simulink model "small_perturbation_linearized_model_v2"  (R2019b)
settings: Solver=ode4  StartTime=0.0  StopTime=20  FixedStep=1e-3
settings Model: Creator=bitgar  LastModifiedBy=zczhu

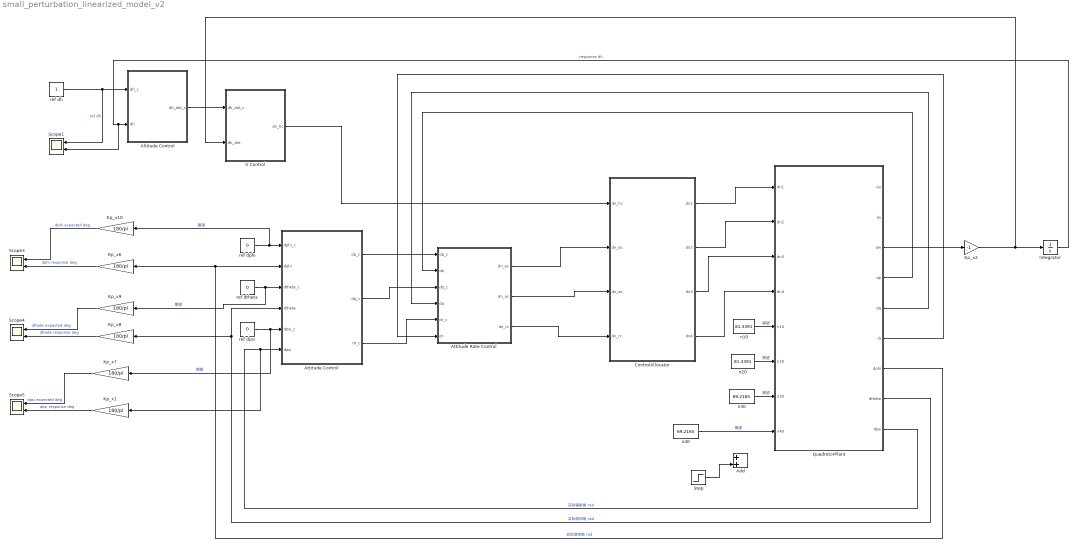
== system small_perturbation_linearized_model_v2 ==
  Add : Sum
  Altitude Control : Subsystem
  Attitude Control : Subsystem
  Attitude Rate Control : Subsystem
  ControlAllocator : Subsystem
  Integrator : Integrator
  Kp_x{1,6..10} (6 alike) : Gain  Gain=180/pi
  Kp_x2 : Gain  Gain=-1
  QuadrotorPlant : Subsystem
  Scope{1,3..5} (4 alike) : Scope  NumInputPorts=2
  Step : Step  Time=5  After=20  SampleTime=0
  V Control : Subsystem
  n10 : Constant  Value=81.3391
  n20 : Constant  Value=81.3391
  n30 : Constant  Value=69.2165
  n40 : Constant  Value=69.2165
  ref dh : Constant
  ref dphi : Constant  Value=0
  ref dpsi : Constant  Value=0
  ref dtheta : Constant  Value=0
  wires:
  Attitude Control/2(dq_c) -> Attitude Rate Control/3(dq_c)
  Attitude Control/1(dp_c) -> Attitude Rate Control/1(dp_c)
  ref dpsi/1 -> Kp_x7/1, Attitude Control/5(dpsi_c)  "期望"
  Attitude Rate Control/2(dn_ac) -> ControlAllocator/3(dn_ac)
  Attitude Rate Control/1(dn_ec) -> ControlAllocator/2(dn_ec)
  Attitude Rate Control/3(dn_rc) -> ControlAllocator/4(dn_rc)
  Attitude Control/3(dr_c) -> Attitude Rate Control/5(dr_c)
  Kp_x6/1 -> Scope3/2  "dphi response deg"
  Kp_x8/1 -> Scope4/2  "dtheta response deg"
  ControlAllocator/2(dn2) -> QuadrotorPlant/2(dn2)
  ControlAllocator/3(dn3) -> QuadrotorPlant/3(dn3)
  ControlAllocator/4(dn4) -> QuadrotorPlant/4(dn4)
  QuadrotorPlant/4(dp) -> Attitude Rate Control/2(dp)
  QuadrotorPlant/5(dq) -> Attitude Rate Control/4(dq)
  QuadrotorPlant/6(dr) -> Attitude Rate Control/6(dr)
  QuadrotorPlant/7(dphi) -> Kp_x6/1, Attitude Control/2(dphi)  "实际滚转角 rad"
  QuadrotorPlant/8(dtheta) -> Kp_x8/1, Attitude Control/4(dtheta)  "实际俯仰角 rad"
  QuadrotorPlant/9(dpsi) -> Kp_x1/1, Attitude Control/6(dpsi)  "实际偏航角 rad"
  ref dphi/1 -> Kp_x10/1, Attitude Control/1(dphi_c)  "期望"
  ref dtheta/1 -> Kp_x9/1, Attitude Control/3(dtheta_c)  "期望"
  n10/1 -> QuadrotorPlant/5(n10)  "期望"
  n20/1 -> QuadrotorPlant/6(n20)  "期望"
  n30/1 -> QuadrotorPlant/7(n30)  "期望"
  Kp_x1/1 -> Scope5/2  "dpsi response deg"
  Kp_x7/1 -> Scope5/1  "dpsi expected deg"
  Kp_x9/1 -> Scope4/1  "dtheta expected deg"
  Kp_x10/1 -> Scope3/1  "dphi expected deg"
  ControlAllocator/1(dn1) -> QuadrotorPlant/1(dn1)
  Step/1 -> Add/2
  ref dh/1 -> Scope1/1, Altitude Control/1(dh_c)  "ref dh"
  Altitude Control/1(dh_dot_c) -> V Control/1(dh_dot_c)
  V Control/1(dn_hc) -> ControlAllocator/1(dn_hc)
  QuadrotorPlant/3(dw) -> Kp_x2/1
  Integrator/1 -> Scope1/2, Altitude Control/2(dh)  "response dh"
  Kp_x2/1 -> V Control/2(dh_dot), Integrator/1
  n40/1 -> QuadrotorPlant/8(n40)  "期望"

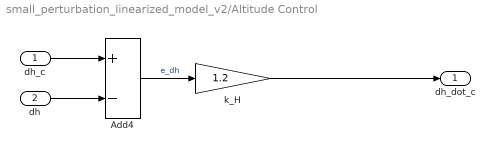
== system small_perturbation_linearized_model_v2/Altitude Control ==
  dh_c : Inport
  dh : Inport  Port=2
  Add4 : Sum  Inputs=+-
  k_H : Gain  Gain=1.2
  dh_dot_c : Outport
  wires:
  dh_c/1 -> Add4/1
  dh/1 -> Add4/2
  Add4/1 -> k_H/1  "e_dh"
  k_H/1 -> dh_dot_c/1

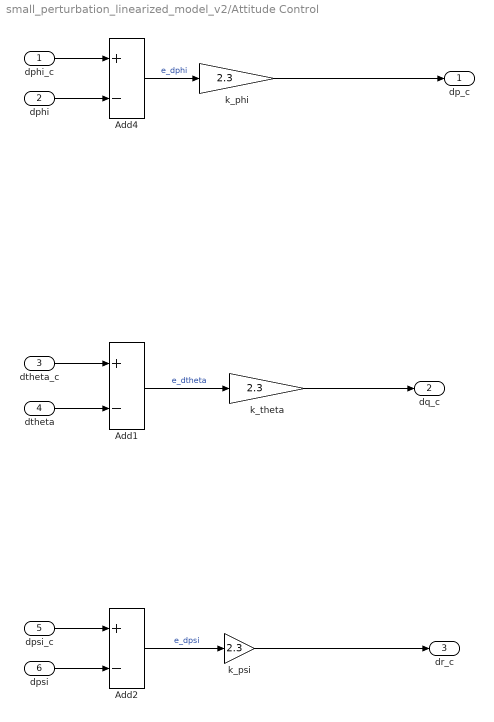
== system small_perturbation_linearized_model_v2/Attitude Control ==
  dphi_c : Inport
  dphi : Inport  Port=2
  dtheta_c : Inport  Port=3
  dtheta : Inport  Port=4
  dpsi_c : Inport  Port=5
  dpsi : Inport  Port=6
  Add1 : Sum  Inputs=+-
  Add2 : Sum  Inputs=+-
  Add4 : Sum  Inputs=+-
  k_phi : Gain  Gain=2.3
  k_psi : Gain  Gain=2.3
  k_theta : Gain  Gain=2.3
  dp_c : Outport
  dq_c : Outport  Port=2
  dr_c : Outport  Port=3
  wires:
  dphi_c/1 -> Add4/1
  dphi/1 -> Add4/2
  dtheta_c/1 -> Add1/1
  dtheta/1 -> Add1/2
  dpsi/1 -> Add2/2
  Add4/1 -> k_phi/1  "e_dphi"
  dpsi_c/1 -> Add2/1
  Add1/1 -> k_theta/1  "e_dtheta"
  Add2/1 -> k_psi/1  "e_dpsi"
  k_phi/1 -> dp_c/1
  k_theta/1 -> dq_c/1
  k_psi/1 -> dr_c/1

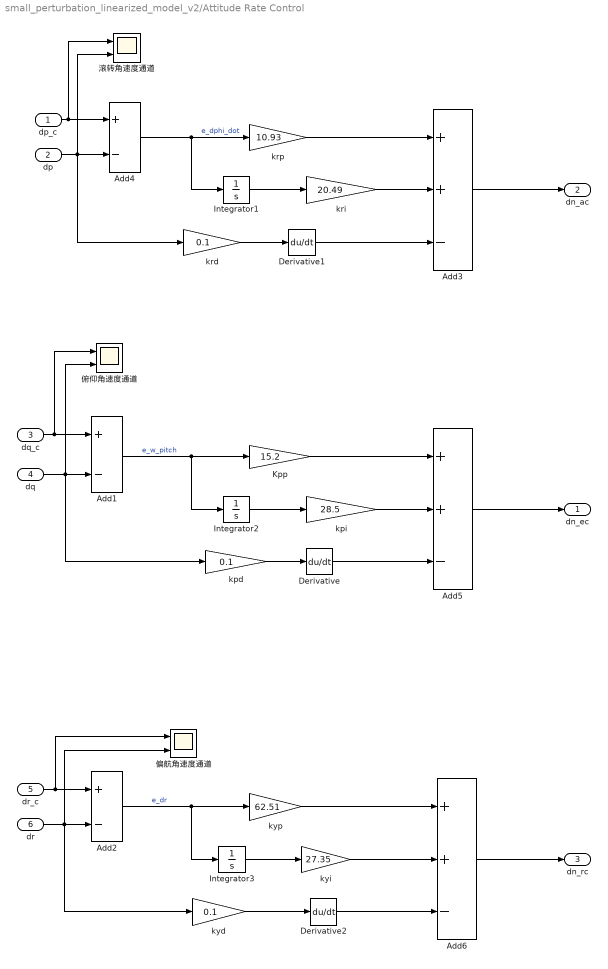
== system small_perturbation_linearized_model_v2/Attitude Rate Control ==
  dp_c : Inport
  dp : Inport  Port=2
  dq_c : Inport  Port=3
  dq : Inport  Port=4
  dr_c : Inport  Port=5
  dr : Inport  Port=6
  Add1 : Sum  Inputs=+-
  Add2 : Sum  Inputs=+-
  Add3 : Sum  Inputs=++-
  Add4 : Sum  Inputs=+-
  Add5 : Sum  Inputs=++-
  Add6 : Sum  Inputs=++-
  Derivative : Derivative
  Derivative1 : Derivative
  Derivative2 : Derivative
  Integrator1 : Integrator
  Integrator2 : Integrator
  Integrator3 : Integrator
  Kpp : Gain  Gain=15.2
  kpd : Gain  Gain=0.1
  kpi : Gain  Gain=28.5
  krd : Gain  Gain=0.1
  kri : Gain  Gain=20.49
  krp : Gain  Gain=10.93
  kyd : Gain  Gain=0.1
  kyi : Gain  Gain=27.35
  kyp : Gain  Gain=62.51
  俯仰角速度通道 : Scope  NumInputPorts=2
  偏航角速度通道 : Scope  NumInputPorts=2
  滚转角速度通道 : Scope  NumInputPorts=2
  dn_ec : Outport
  dn_ac : Outport  Port=2
  dn_rc : Outport  Port=3
  wires:
  dp_c/1 -> 滚转角速度通道/1, Add4/1
  dp/1 -> krd/1, 滚转角速度通道/2, Add4/2
  dq_c/1 -> 俯仰角速度通道/1, Add1/1
  dq/1 -> kpd/1, 俯仰角速度通道/2, Add1/2
  dr/1 -> 偏航角速度通道/2, kyd/1, Add2/2
  Add4/1 -> Integrator1/1, krp/1  "e_dphi_dot"
  dr_c/1 -> 偏航角速度通道/1, Add2/1
  Add3/1 -> dn_ac/1
  kri/1 -> Add3/2
  krp/1 -> Add3/1
  Integrator1/1 -> kri/1
  Integrator2/1 -> kpi/1
  Kpp/1 -> Add5/1
  kpi/1 -> Add5/2
  Add1/1 -> Integrator2/1, Kpp/1  "e_w_pitch"
  Add5/1 -> dn_ec/1
  Add2/1 -> Integrator3/1, kyp/1  "e_dr"
  Integrator3/1 -> kyi/1
  kyp/1 -> Add6/1
  kyi/1 -> Add6/2
  Add6/1 -> dn_rc/1
  kpd/1 -> Derivative/1
  Derivative/1 -> Add5/3
  krd/1 -> Derivative1/1
  Derivative1/1 -> Add3/3
  kyd/1 -> Derivative2/1
  Derivative2/1 -> Add6/3

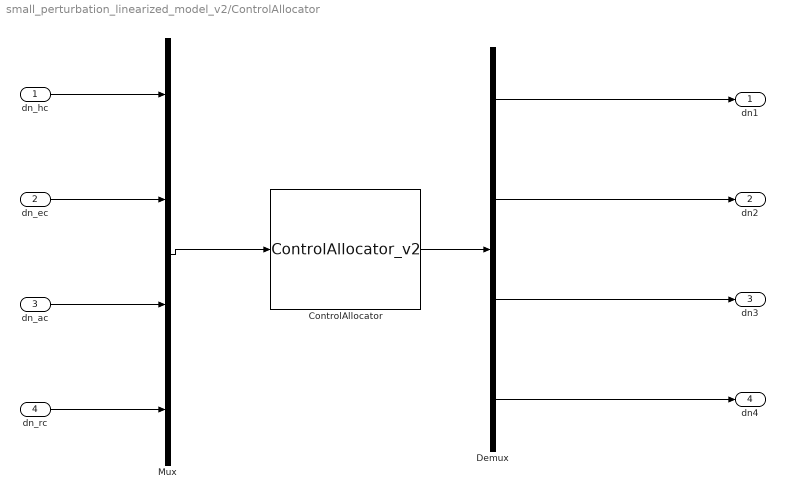
== system small_perturbation_linearized_model_v2/ControlAllocator ==
  dn_hc : Inport
  dn_ec : Inport  Port=2
  dn_ac : Inport  Port=3
  dn_rc : Inport  Port=4
  ControlAllocator : S-Function  FunctionName=ControlAllocator_v2  SFunctionDeploymentMode=off  EnableBusSupport=off
  Demux : Demux
  Mux : Mux
  dn1 : Outport
  dn2 : Outport  Port=2
  dn3 : Outport  Port=3
  dn4 : Outport  Port=4
  wires:
  Demux/2 -> dn2/1
  Demux/1 -> dn1/1
  Demux/3 -> dn3/1
  Demux/4 -> dn4/1
  Mux/1 -> ControlAllocator/1
  dn_ec/1 -> Mux/2
  dn_ac/1 -> Mux/3
  dn_rc/1 -> Mux/4
  ControlAllocator/1 -> Demux/1
  dn_hc/1 -> Mux/1

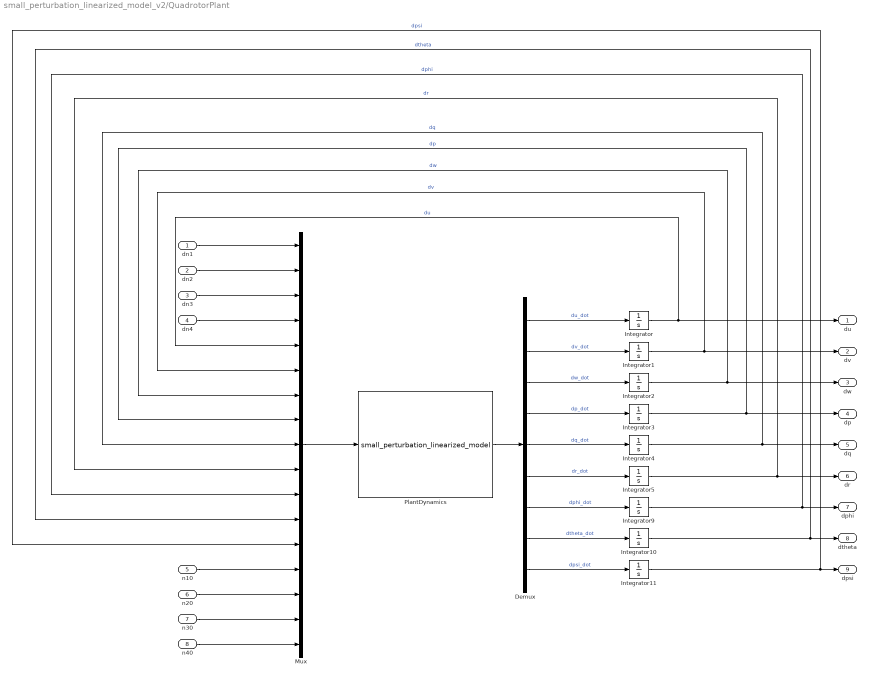
== system small_perturbation_linearized_model_v2/QuadrotorPlant ==
  dn1 : Inport
  dn2 : Inport  Port=2
  dn3 : Inport  Port=3
  dn4 : Inport  Port=4
  n10 : Inport  Port=5
  n20 : Inport  Port=6
  n30 : Inport  Port=7
  n40 : Inport  Port=8
  Demux : Demux  Outputs=9
  Integrator{,1..5,9..11} (9 alike) : Integrator
  Mux : Mux  Inputs=17
  PlantDynamics : S-Function  FunctionName=small_perturbation_linearized_model  Parameters=1 9.81 21 29 55 45 0.00043 0.00078 0.01239 0.01239 0.02382 0  SFunctionDeploymentMode=off  EnableBusSupport=off
  du : Outport
  dv : Outport  Port=2
  dw : Outport  Port=3
  dp : Outport  Port=4
  dq : Outport  Port=5
  dr : Outport  Port=6
  dphi : Outport  Port=7
  dtheta : Outport  Port=8
  dpsi : Outport  Port=9
  wires:
  Demux/4 -> Integrator3/1  "dp_dot"
  Mux/1 -> PlantDynamics/1
  Demux/3 -> Integrator2/1  "dw_dot"
  dn2/1 -> Mux/2
  Demux/1 -> Integrator/1  "du_dot"
  Demux/5 -> Integrator4/1  "dq_dot"
  Demux/6 -> Integrator5/1  "dr_dot"
  Demux/2 -> Integrator1/1  "dv_dot"
  dn4/1 -> Mux/4
  dn1/1 -> Mux/1
  dn3/1 -> Mux/3
  PlantDynamics/1 -> Demux/1
  Integrator9/1 -> Mux/11, dphi/1  "dphi"
  Integrator10/1 -> Mux/12, dtheta/1  "dtheta"
  Integrator11/1 -> Mux/13, dpsi/1  "dpsi"
  Integrator/1 -> du/1, Mux/5  "du"
  Integrator1/1 -> Mux/6, dv/1  "dv"
  Integrator2/1 -> Mux/7, dw/1  "dw"
  Demux/7 -> Integrator9/1  "dphi_dot"
  Demux/8 -> Integrator10/1  "dtheta_dot"
  Demux/9 -> Integrator11/1  "dpsi_dot"
  Integrator3/1 -> Mux/8, dp/1  "dp"
  Integrator4/1 -> Mux/9, dq/1  "dq"
  Integrator5/1 -> Mux/10, dr/1  "dr"
  n30/1 -> Mux/16
  n10/1 -> Mux/14
  n20/1 -> Mux/15
  n40/1 -> Mux/17

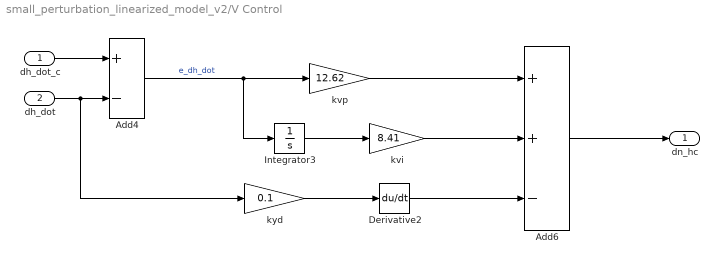
== system small_perturbation_linearized_model_v2/V Control ==
  dh_dot_c : Inport
  dh_dot : Inport  Port=2
  Add4 : Sum  Inputs=+-
  Add6 : Sum  Inputs=++-
  Derivative2 : Derivative
  Integrator3 : Integrator
  kvi : Gain  Gain=8.41
  kvp : Gain  Gain=12.62
  kyd : Gain  Gain=0.1
  dn_hc : Outport
  wires:
  dh_dot_c/1 -> Add4/1
  dh_dot/1 -> kyd/1, Add4/2
  Add4/1 -> Integrator3/1, kvp/1  "e_dh_dot"
  Derivative2/1 -> Add6/3
  kyd/1 -> Derivative2/1
  Add6/1 -> dn_hc/1
  kvi/1 -> Add6/2
  Integrator3/1 -> kvi/1
  kvp/1 -> Add6/1
